simulink model "thrust_curve_import_test"  (R2014a)
settings: Solver=ode3  StartTime=0.0  StopTime=10.0  FixedStep=0.01  RelTol=1e-3
libraries: rocket_dynamic_data_library x1, simulink x1
settings Model: Creator=scorpii  LastModifiedBy=scorpii

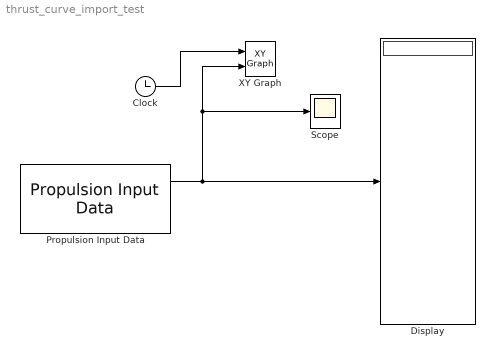
== system thrust_curve_import_test ==
  Clock : Clock
  Display : Display
  Propulsion Input Data : rocket_dynamic_data_library/Propulsion Input Data
  Scope : Scope
      settings: YMin=0  YMax=2500
  XY Graph : simulink/Sinks/XY Graph  xmin=0  xmax=4.4  ymin=0  ymax=2500  st=-1
  wires:
  Propulsion Input Data/1 -> Display/1, Scope/1, XY Graph/2
  Clock/1 -> XY Graph/1
